simulink model "SMC"  (R2022b)
settings: Solver=VariableStepAuto  StartTime=0.0  StopTime=10.0  RelTol=1e-3
settings Model: Creator=hollis  LastModifiedBy=hollis

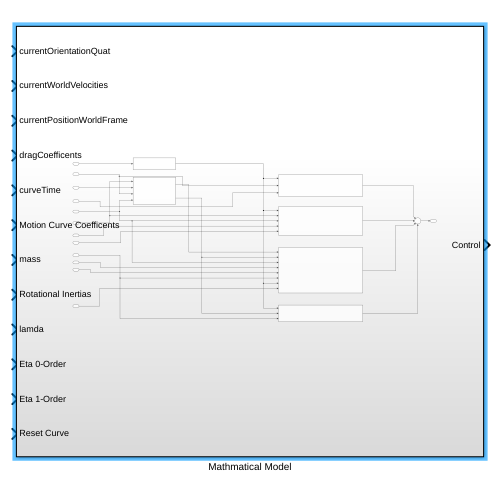
[thumbnail: Simulink's stored preview of the top-level diagram]
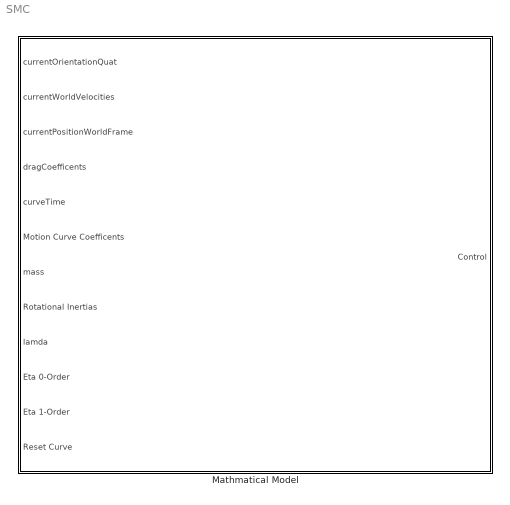
== system SMC ==
  Mathmatical Model : Subsystem

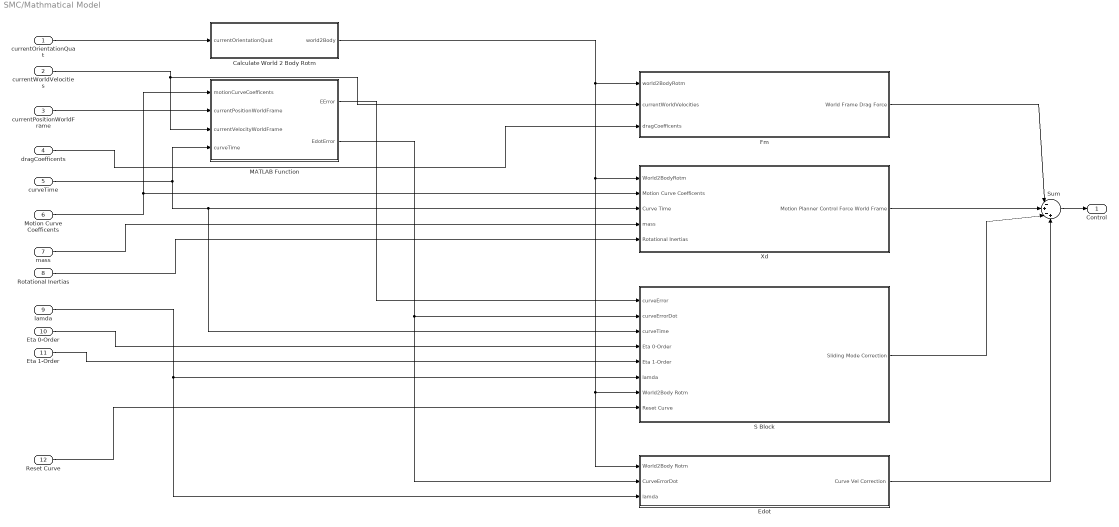
== system SMC/Mathmatical Model ==
  currentOrientationQuat : Inport
  currentWorldVelocities : Inport  Port=2
  currentPositionWorldFrame : Inport  Port=3
  dragCoefficents : Inport  Port=4
  curveTime : Inport  Port=5
  Motion Curve Coefficents : Inport  Port=6
  mass : Inport  Port=7
  Rotational Inertias : Inport  Port=8
  lamda : Inport  Port=9
  Eta 0-Order : Inport  Port=10
  Eta 1-Order : Inport  Port=11
  Reset Curve : Inport  Port=12
  Calculate World 2 Body Rotm : MATLAB Function  TreatAsAtomicUnit=on
  Edot : Subsystem
  Fm : Subsystem
  MATLAB Function : MATLAB Function  TreatAsAtomicUnit=on
  S Block : Subsystem
  Sum : Sum  Inputs=|-+-+
  Xd : Subsystem
  Control : Outport
  wires:
  Reset Curve/1 -> S Block/8(Reset Curve)
  Eta 0-Order/1 -> S Block/4(Eta 0-Order)
  Eta 1-Order/1 -> S Block/5(Eta 1-Order)
  currentWorldVelocities/1 -> MATLAB Function/3(currentVelocityWorldFrame), Fm/2(currentWorldVelocities)
  MATLAB Function/2(EdotError) -> Edot/2(CurveErrorDot), S Block/2(curveErrorDot)
  Fm/1(World Frame Drag Force) -> Sum/1
  mass/1 -> Xd/4(mass)
  Motion Curve Coefficents/1 -> Xd/2(Motion Curve Coefficents), MATLAB Function/1(motionCurveCoefficents)
  currentPositionWorldFrame/1 -> MATLAB Function/2(currentPositionWorldFrame)
  dragCoefficents/1 -> Fm/3(dragCoefficents)
  curveTime/1 -> MATLAB Function/4(curveTime), S Block/3(curveTime), Xd/3(Curve Time)
  Xd/1(Motion Planner Control Force World Frame) -> Sum/2
  MATLAB Function/1(EError) -> S Block/1(curveError)
  S Block/1("Sliding Mode Correction ") -> Sum/3
  lamda/1 -> Edot/3(lamda), S Block/6(lamda)
  Rotational Inertias/1 -> Xd/5(Rotational Inertias)
  Calculate World 2 Body Rotm/1(world2Body) -> Edot/1(World2Body Rotm), S Block/7(World2Body Rotm), Xd/1(World2BodyRotm), Fm/1(world2BodyRotm)
  currentOrientationQuat/1 -> Calculate World 2 Body Rotm/1(currentOrientationQuat)
  Edot/1(Curve Vel Correction) -> Sum/4
  Sum/1 -> Control/1

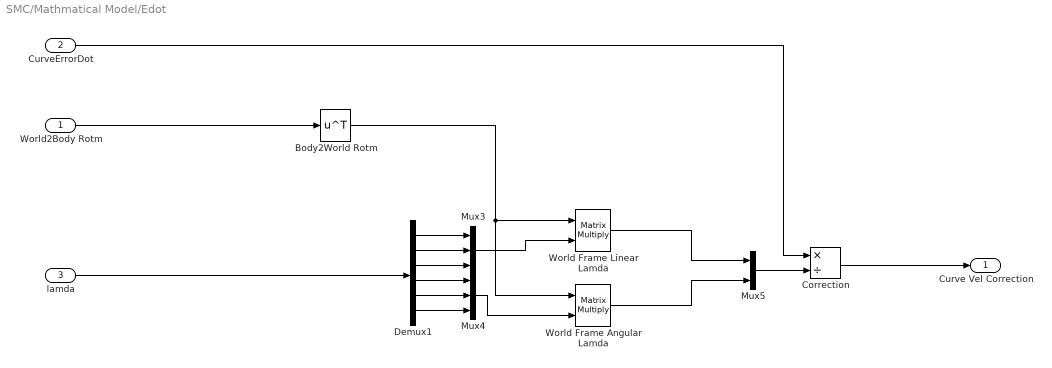
== system SMC/Mathmatical Model/Edot ==
  World2Body Rotm : Inport
  CurveErrorDot : Inport  Port=2
  lamda : Inport  Port=3
  Body2World Rotm : Math  Operator=transpose
  Correction : Product  Inputs=*/
  Demux1 : Demux  Outputs=6
  Mux3 : Mux  Inputs=3
  Mux4 : Mux  Inputs=3
  Mux5 : Mux  Inputs=2
  World Frame Angular Lamda : Product  Multiplication=Matrix(*)
  World Frame Linear Lamda : Product  Multiplication=Matrix(*)
  Curve Vel Correction : Outport
  wires:
  Demux1/5 -> Mux4/2
  Mux3/1 -> World Frame Linear Lamda/2
  Demux1/6 -> Mux4/3
  CurveErrorDot/1 -> Correction/1
  Body2World Rotm/1 -> World Frame Angular Lamda/1, World Frame Linear Lamda/1
  World2Body Rotm/1 -> Body2World Rotm/1
  Mux4/1 -> World Frame Angular Lamda/2
  World Frame Angular Lamda/1 -> Mux5/2
  Demux1/4 -> Mux4/1
  Demux1/3 -> Mux3/3
  World Frame Linear Lamda/1 -> Mux5/1
  Correction/1 -> Curve Vel Correction/1
  Demux1/1 -> Mux3/1
  lamda/1 -> Demux1/1
  Mux5/1 -> Correction/2
  Demux1/2 -> Mux3/2

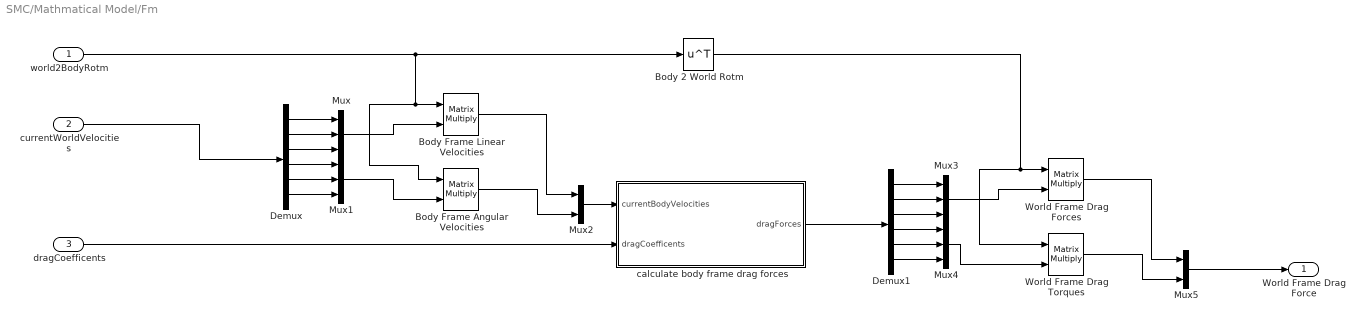
== system SMC/Mathmatical Model/Fm ==
  world2BodyRotm : Inport
  currentWorldVelocities : Inport  Port=2
  dragCoefficents : Inport  Port=3
  Body 2 World Rotm : Math  Operator=transpose
  Body Frame Angular Velocities : Product  Multiplication=Matrix(*)
  Body Frame Linear Velocities : Product  Multiplication=Matrix(*)
  Demux : Demux  Outputs=6
  Demux1 : Demux  Outputs=6
  Mux{,1,3..4} (4 alike) : Mux  Inputs=3
  Mux2 : Mux  Inputs=2
  Mux5 : Mux  Inputs=2
  World Frame Drag Forces : Product  Multiplication=Matrix(*)
  World Frame Drag Torques : Product  Multiplication=Matrix(*)
  calculate body frame drag forces : MATLAB Function  TreatAsAtomicUnit=on
  World Frame Drag Force : Outport
  wires:
  Body Frame Linear Velocities/1 -> Mux2/1
  World Frame Drag Forces/1 -> Mux5/1
  Demux1/4 -> Mux4/1
  Demux1/1 -> Mux3/1
  Mux/1 -> Body Frame Linear Velocities/2
  Mux3/1 -> World Frame Drag Forces/2
  Demux1/3 -> Mux3/3
  Demux1/6 -> Mux4/3
  Mux5/1 -> World Frame Drag Force/1
  currentWorldVelocities/1 -> Demux/1
  Mux1/1 -> Body Frame Angular Velocities/2
  Demux/4 -> Mux1/1
  Demux/3 -> Mux/3
  Demux1/2 -> Mux3/2
  World Frame Drag Torques/1 -> Mux5/2
  Mux2/1 -> calculate body frame drag forces/1(currentBodyVelocities)
  dragCoefficents/1 -> calculate body frame drag forces/2(dragCoefficents)
  Demux/5 -> Mux1/2
  Demux/2 -> Mux/2
  Demux1/5 -> Mux4/2
  Demux/6 -> Mux1/3
  world2BodyRotm/1 -> Body Frame Angular Velocities/1, Body Frame Linear Velocities/1, Body 2 World Rotm/1
  Mux4/1 -> World Frame Drag Torques/2
  Demux/1 -> Mux/1
  Body 2 World Rotm/1 -> World Frame Drag Torques/1, World Frame Drag Forces/1
  Body Frame Angular Velocities/1 -> Mux2/2
  calculate body frame drag forces/1(dragForces) -> Demux1/1

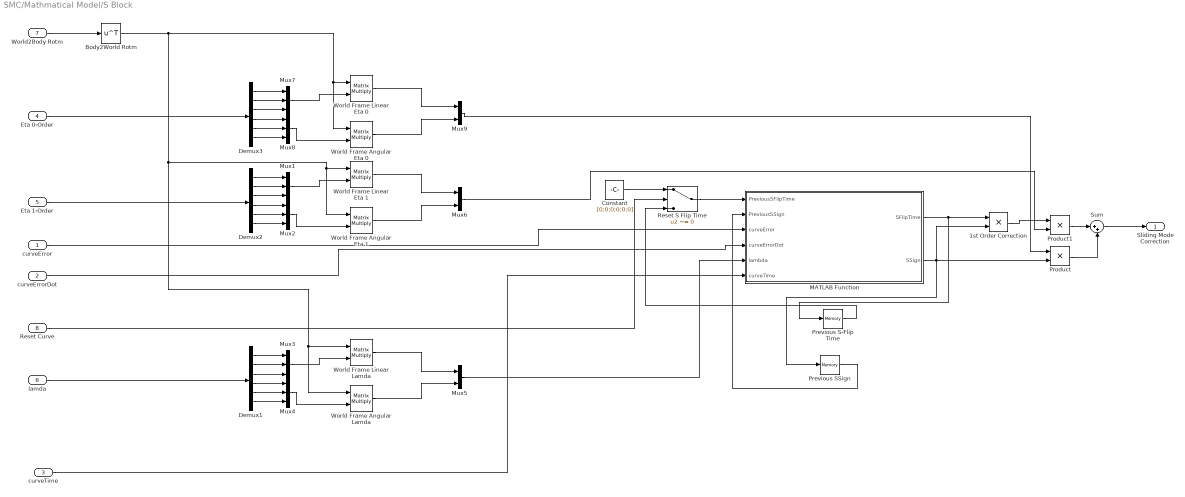
== system SMC/Mathmatical Model/S Block ==
  curveError : Inport
  curveErrorDot : Inport  Port=2
  curveTime : Inport  Port=3
  Eta 0-Order : Inport  Port=4
  Eta 1-Order : Inport  Port=5
  lamda : Inport  Port=6
  World2Body Rotm : Inport  Port=7
  Reset Curve : Inport  Port=8
  1st Order Correction : Product
  Body2World Rotm : Math  Operator=transpose
  Constant : Constant  Value=[0;0;0;0;0;0]
  Demux1 : Demux  Outputs=6
  Demux2 : Demux  Outputs=6
  Demux3 : Demux  Outputs=6
  MATLAB Function : MATLAB Function  TreatAsAtomicUnit=on
  Mux{1..4,7..8} (6 alike) : Mux  Inputs=3
  Mux5 : Mux  Inputs=2
  Mux6 : Mux  Inputs=2
  Mux9 : Mux  Inputs=2
  Previous S-Flip Time : Memory  InitialCondition=[0;0;0;0;0;0]
  Previous SSign : Memory  InitialCondition=[1;1;1;1;1;1]
  Product : Product
  Product1 : Product
  Reset S Flip Time : Switch  Criteria=u2 ~= 0  SaturateOnIntegerOverflow=off  InputSameDT=off
  Sum : Sum  Inputs=|++
  World Frame Angular Eta 0 : Product  Multiplication=Matrix(*)
  World Frame Angular Eta 1 : Product  Multiplication=Matrix(*)
  World Frame Angular Lamda : Product  Multiplication=Matrix(*)
  World Frame Linear Eta 0 : Product  Multiplication=Matrix(*)
  World Frame Linear Eta 1 : Product  Multiplication=Matrix(*)
  World Frame Linear Lamda : Product  Multiplication=Matrix(*)
  "Sliding Mode Correction " : Outport
  wires:
  Previous SSign/1 -> MATLAB Function/2(PreviousSSign)
  Mux5/1 -> MATLAB Function/5(lambda)
  MATLAB Function/2(SSign) -> 1st Order Correction/2, Product/2, Previous SSign/1
  curveTime/1 -> MATLAB Function/6(curveTime)
  MATLAB Function/1(SFlipTime) -> 1st Order Correction/1, Previous S-Flip Time/1
  curveErrorDot/1 -> MATLAB Function/4(curveErrorDot)
  curveError/1 -> MATLAB Function/3(curveError)
  Product/1 -> Sum/2
  Product1/1 -> Sum/1
  1st Order Correction/1 -> Product1/1
  Sum/1 -> "Sliding Mode Correction "/1
  Demux1/1 -> Mux3/1
  Demux1/2 -> Mux3/2
  lamda/1 -> Demux1/1
  Demux1/5 -> Mux4/2
  Demux1/3 -> Mux3/3
  Demux1/6 -> Mux4/3
  Mux3/1 -> World Frame Linear Lamda/2
  World Frame Linear Lamda/1 -> Mux5/1
  World Frame Angular Lamda/1 -> Mux5/2
  Demux1/4 -> Mux4/1
  Mux4/1 -> World Frame Angular Lamda/2
  Demux2/1 -> Mux1/1
  Demux2/4 -> Mux2/1
  Demux2/5 -> Mux2/2
  Demux2/2 -> Mux1/2
  Demux2/6 -> Mux2/3
  Demux2/3 -> Mux1/3
  World Frame Linear Eta 1/1 -> Mux6/1
  Mux1/1 -> World Frame Linear Eta 1/2
  Mux2/1 -> World Frame Angular Eta 1/2
  World Frame Angular Eta 1/1 -> Mux6/2
  Body2World Rotm/1 -> World Frame Linear Eta 1/1, World Frame Angular Eta 1/1, World Frame Linear Lamda/1, World Frame Angular Lamda/1, World Frame Angular Eta 0/1, World Frame Linear Eta 0/1
  Eta 1-Order/1 -> Demux2/1
  Mux6/1 -> Product1/2
  Mux8/1 -> World Frame Angular Eta 0/2
  Demux3/2 -> Mux7/2
  Demux3/3 -> Mux7/3
  Eta 0-Order/1 -> Demux3/1
  Demux3/6 -> Mux8/3
  Demux3/1 -> Mux7/1
  Demux3/4 -> Mux8/1
  World Frame Linear Eta 0/1 -> Mux9/1
  Demux3/5 -> Mux8/2
  Mux9/1 -> Product/1
  World Frame Angular Eta 0/1 -> Mux9/2
  Mux7/1 -> World Frame Linear Eta 0/2
  World2Body Rotm/1 -> Body2World Rotm/1
  Reset S Flip Time/1 -> MATLAB Function/1(PreviousSFlipTime)
  Previous S-Flip Time/1 -> Reset S Flip Time/3
  Constant/1 -> Reset S Flip Time/1
  Reset Curve/1 -> Reset S Flip Time/2

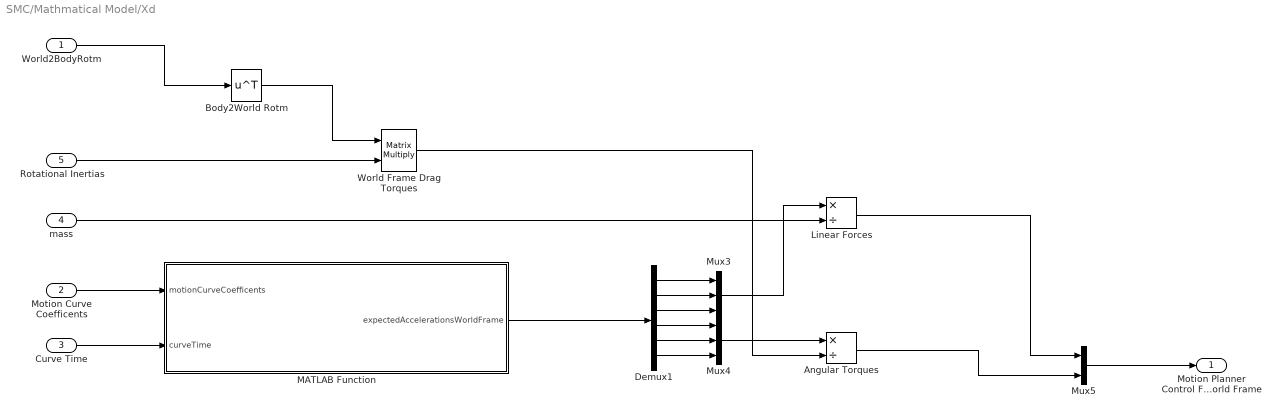
== system SMC/Mathmatical Model/Xd ==
  World2BodyRotm : Inport
  Motion Curve Coefficents : Inport  Port=2
  Curve Time : Inport  Port=3
  mass : Inport  Port=4
  Rotational Inertias : Inport  Port=5
  Angular Torques : Product  Inputs=*/
  Body2World Rotm : Math  Operator=transpose
  Demux1 : Demux  Outputs=6
  Linear Forces : Product  Inputs=*/
  MATLAB Function : MATLAB Function  TreatAsAtomicUnit=on
  Mux3 : Mux  Inputs=3
  Mux4 : Mux  Inputs=3
  Mux5 : Mux  Inputs=2
  World Frame Drag Torques : Product  Multiplication=Matrix(*)
  Motion Planner Control Force World Frame : Outport
  wires:
  Demux1/4 -> Mux4/1
  Curve Time/1 -> MATLAB Function/2(curveTime)
  World2BodyRotm/1 -> Body2World Rotm/1
  Motion Curve Coefficents/1 -> MATLAB Function/1(motionCurveCoefficents)
  Demux1/6 -> Mux4/3
  Demux1/5 -> Mux4/2
  Demux1/3 -> Mux3/3
  Demux1/2 -> Mux3/2
  Mux5/1 -> Motion Planner Control Force World Frame/1
  Demux1/1 -> Mux3/1
  MATLAB Function/1(expectedAccelerationsWorldFrame) -> Demux1/1
  Mux3/1 -> Linear Forces/1
  mass/1 -> Linear Forces/2
  Body2World Rotm/1 -> World Frame Drag Torques/1
  Rotational Inertias/1 -> World Frame Drag Torques/2
  Mux4/1 -> Angular Torques/1
  World Frame Drag Torques/1 -> Angular Torques/2
  Angular Torques/1 -> Mux5/2
  Linear Forces/1 -> Mux5/1

== matlab function SMC/Mathmatical Model/Calculate World 2 Body Rotm ==
  data: currentOrientationQuat input; world2Body output
function world2Body = fcn(currentOrientationQuat)

%convert ros2 quat to matlab quat
quat = [currentOrientationQuat(4), currentOrientationQuat(1), currentOrientationQuat(2), currentOrientationQuat(3)];

%calculate the rotation matrix representing the current orientation
world2Body = quat2rotm(quat);

== matlab function SMC/Mathmatical Model/Fm/calculate body frame drag forces ==
  data: currentBodyVelocities input; dragForces output; dragCoefficents input
function dragForces = fcn(currentBodyVelocities, dragCoefficents)

dragForces = zeros(6,1);

expectedDragCoefficentLength = 18;
if(expectedDragCoefficentLength ~= length(dragCoefficents))
    %drag coefficents are not the expected length
    return 
end

%reshape drag coefficents array into a more sensible form
dc = reshape(dragCoefficents, [6, expectedDragCoefficentLength / 6]);

for i=1:6
    %calculate the forces created by drag
    dragForces(i) = currentBodyVelocities(i) * dc(i, 2) + currentBodyVelocities(i) ^ 2 * dc(i, 3) + dc(i, 1);
end

== matlab function SMC/Mathmatical Model/Xd/MATLAB Function ==
  data: motionCurveCoefficents input; expectedAccelerationsWorldFrame output; curveTime input
function expectedAccelerationsWorldFrame = fcn(motionCurveCoefficents, curveTime)

%default values for the expected accelerations in world frame
expectedAccelerationsWorldFrame = zeros(6,1);

expectedCurveCofficents = 18;
if(expectedCurveCofficents ~= sum(size(motionCurveCoefficents)))
    %ensure expected number of curve coefficents are delivered
    return
end

for i = 1:6
    %calculate expectedAccelerations for each dof
    %these curves should be the double derivative of the motion planner
    %curves
    expectedAccelerationsWorldFrame = -sin(2 * pi() * curveTime) * k(3) * 4 * pi()^2;
end

== matlab function SMC/Mathmatical Model/S Block/MATLAB Function ==
  data: PreviousSFlipTime input; SFlipTime output; PreviousSSign input; curveError input; curveErrorDot input; lambda input; curveTime input; SSign output
function [SFlipTime, SSign] = fcn(PreviousSFlipTime, PreviousSSign, curveError, curveErrorDot, lambda, curveTime)

%FlipTime, SSign and Previous are 6 by arrays - 1 per dof

SFlipTime = PreviousSFlipTime;

%calculate S
S = curveError - lambda * curveErrorDot;

%just so nothing explodes - ill be impressed if this happens
for i=1:6
    %ensure no S equals zero
    if(S(i) == 0)
        S(i) = .0000001;
    end
end

%get S signs as 1 or -1
SSign = S / abs(S);

%see if S has flipped
for i=1:6
    if(SSign(i) * PreviousSSign(i) < 0)
        %S has flipped in dof i
        SFlipTime(i) = curveTime;
    end
end

== matlab function SMC/Mathmatical Model/MATLAB Function ==
  data: motionCurveCoefficents input; EError output; currentPositionWorldFrame input; currentVelocityWorldFrame input; curveTime input; EdotError output
function [EError, EdotError] = fcn(motionCurveCoefficents, currentPositionWorldFrame, currentVelocityWorldFrame, curveTime)

%current position world frame and current velocity world frame are six * 1
%vectors

%default values
EError = zeros(6,1);
EdotError = zeros(6,1);

expectedMotionCurveCoefficents = 18;
if(expectedMotionCurveCoefficents ~= sum(size(motionCurveCoefficents)))
    %inccorect motion curve coefficents
    return
end

%evaulate each dof seperately
for i=1:6
    %calculate motion curve expected position
    curvePos = motionCurveCoefficents(i, 1) + motionCurveCoefficents(i, 2) * curveTime + motionCurveCoefficents(i, 3) * sin(2*pi()*curveTime);
    %calculate motion curve expected velocity
    curveVel = motionCurveCoefficents(i, 2) + motionCurveCoefficents(i, 3) * cos(2*pi()*curveTime) * 2 * pi();

    %calculate position error
    if(i <= 3)
        EError(i) = currentPositionWorldFrame(i) - curvePos(i);
    else
        %for angular error - need to compensate for loop around
        EError(i) = currentPositionWorldFrame(i) - curvePos(i);

        %normalize Error to 0 to 2pi
        EError(i) = mod(EError(i), 2 * pi());

        %if error greater than pi - smaller error in negative direction
        if(EError(i) > pi())
            EError(i) = EError(i) - 2 * pi();
        end
    end

    %calculate velocity error
    EdotError(i) = currentVelocityWorldFrame(i) - curveVel(i);
end
